simulink model "FSAC2021_V1"  (R2014a)
settings: Solver=FixedStepDiscrete  StartTime=0.0  StopTime=inf  FixedStep=0.0005  RelTol=1e-3
model workspace (MAT data in the model file):
  AS_READY = Simulink.Parameter
  AS_READY.Value = 2
  AS_READY.DataType = 'uint8'
  AS_DRIVING = Simulink.Parameter
  AS_DRIVING.Value = 3
  AS_DRIVING.DataType = 'uint8'
  AS_OFF = Simulink.Parameter
  AS_OFF.Value = 1
  AS_OFF.DataType = 'uint8'
  AS_FINISH = Simulink.Parameter
  AS_FINISH.Value = 4
  AS_FINISH.DataType = 'uint8'
  AS_EMERGENCY = Simulink.Parameter
  AS_EMERGENCY.Value = 5
  AS_EMERGENCY.DataType = 'uint8'
  ENABLE = Simulink.Parameter
  ENABLE.Value = 1
  ENABLE.DataType = 'uint8'
  DISABLE = Simulink.Parameter
  DISABLE.Value = 0
  DISABLE.DataType = 'uint8'
  Tire_Radius = Simulink.Parameter
  Tire_Radius.Value = 234
  Tire_Radius.DataType = 'single'
  Ts = Simulink.Parameter
  Ts.Value = 0.0005
  Ts.DataType = 'double'
  Filter_Factor = Simulink.Parameter
  Filter_Factor.Value = 0.5
  Filter_Factor.DataType = 'single'
  Teeth_Wheel = Simulink.Parameter
  Teeth_Wheel.Value = 60
  Teeth_Wheel.DataType = 'uint8'
  BLINK = Simulink.Parameter
  BLINK.Value = 2
  BLINK.DataType = 'uint8'
  OFF = Simulink.Parameter
  OFF.Value = 0
  OFF.DataType = 'uint8'
  ON = Simulink.Parameter
  ON.Value = 1
  ON.DataType = 'uint8'
  EBS_DISABLE = Simulink.Parameter
  EBS_DISABLE.Value = 0
  EBS_DISABLE.DataType = 'uint8'
  EBS_ARMED = Simulink.Parameter
  EBS_ARMED.Value = 1
  EBS_ARMED.DataType = 'uint8'
  EBS_ENABLE = Simulink.Parameter
  EBS_ENABLE.Value = 2
  EBS_ENABLE.DataType = 'uint8'
  MANUAL_DRIVING = Simulink.Parameter
  MANUAL_DRIVING.Value = 6
  MANUAL_DRIVING.DataType = 'uint8'
  MANUAL_MODE = Simulink.Parameter
  MANUAL_MODE.Value = 6
  MANUAL_MODE.DataType = 'uint8'
  BUZZER_START = 1
  BUZZER_EBS = Simulink.Parameter
  BUZZER_EBS.Value = 2
  BUZZER_EBS.DataType = 'uint8'
  TRACKDRIVE = Simulink.Parameter
  TRACKDRIVE.Value = 3
  TRACKDRIVE.DataType = 'uint8'
  Self_Learn_Diff = Simulink.Parameter
  Self_Learn_Diff.Value = 150
  Self_Learn_Diff.DataType = 'uint16'
  Acc_Left_Full_mv = Simulink.Parameter
  Acc_Left_Full_mv.Value = 2000
  Acc_Left_Full_mv.DataType = 'single'
  Acc_Right_Full_mv = Simulink.Parameter
  Acc_Right_Full_mv.Value = 2000
  Acc_Right_Full_mv.DataType = 'single'
  Brk_Calib_Value = Simulink.Parameter
  Brk_Calib_Value.Value = 150
  Brk_Calib_Value.DataType = 'single'
  Brk_Use_Range = Simulink.Parameter
  Brk_Use_Range.Value = 1500
  Brk_Use_Range.DataType = 'single'
  Armed = Simulink.Parameter
  Armed.Value = 1
  Armed.DataType = 'uint8'
  Enable = Simulink.Parameter
  Enable.Value = 2
  Enable.DataType = 'uint8'
  Disable = Simulink.Parameter
  Disable.Value = 0
  Disable.DataType = 'uint8'
  High_V = Simulink.Parameter
  High_V.Value = 60
  High_V.DataType = 'uint8'
  reg_num = Simulink.Parameter
  reg_num.Value = 1
  reg_num.DataType = 'uint8'
  Acc_Diff = Simulink.Parameter
  Acc_Diff.Value = 0.3
  Acc_Diff.DataType = 'single'
  Mtr_Cabli = Simulink.Parameter
  Mtr_Cabli.Value = 3
  Mtr_Cabli.DataType = 'single'
  BMS_Cabli = Simulink.Parameter
  BMS_Cabli.Value = 3
  BMS_Cabli.DataType = 'single'
  EBS_Cabli = Simulink.Parameter
  EBS_Cabli.Value = 3.3
  EBS_Cabli.DataType = 'single'
  Acc_Right_Factor = Simulink.Parameter
  Acc_Right_Factor.Value = -0.0833
  Acc_Right_Factor.DataType = 'double'
  Acc_Left_Factor = Simulink.Parameter
  Acc_Left_Factor.Value = 0.045
  Acc_Left_Factor.DataType = 'double'
  Acc_Lft_Offset = Simulink.Parameter
  Acc_Lft_Offset.Value = -90
  Acc_Lft_Offset.DataType = 'int8'
  Acc_Right_Offset = Simulink.Parameter
  Acc_Right_Offset.Value = 408.33
  Acc_Right_Offset.DataType = 'single'
  RTeeth_Wheel = Simulink.Parameter
  RTeeth_Wheel.Value = 30
  RTeeth_Wheel.DataType = 'uint8'
  FTeeth_Wheel = Simulink.Parameter
  FTeeth_Wheel.Value = 60
  FTeeth_Wheel.DataType = 'uint8'
  Brk_Liquid_Prs_Offset = Simulink.Parameter
  Brk_Liquid_Prs_Offset.Value = 0
  Brk_Liquid_Prs_Offset.DataType = 'single'
  Brk_Liquid_Prs_Factor = Simulink.Parameter
  Brk_Liquid_Prs_Factor.Value = 0.001
  Brk_Liquid_Prs_Factor.DataType = 'double'
  EBS_Prs_Factor = Simulink.Parameter
  EBS_Prs_Factor.Value = 0.000303
  EBS_Prs_Factor.DataType = 'double'
  EBS_Prs_Offset = Simulink.Parameter
  EBS_Prs_Offset.Value = 0
  EBS_Prs_Offset.DataType = 'single'
  Mtr_Volt_Factor = Simulink.Parameter
  Mtr_Volt_Factor.Value = 33.33
  Mtr_Volt_Factor.DataType = 'single'
  Mtr_Volt_Offset = Simulink.Parameter
  Mtr_Volt_Offset.Value = 0
  Mtr_Volt_Offset.DataType = 'single'
  BMS_Output_Volt_Factor = Simulink.Parameter
  BMS_Output_Volt_Factor.Value = 33.33
  BMS_Output_Volt_Factor.DataType = 'single'
  BMS_Output_Volt_Offset = Simulink.Parameter
  BMS_Output_Volt_Offset.Value = 0
  BMS_Output_Volt_Offset.DataType = 'single'
  Min = Simulink.Parameter
  Min.Value = 10
  Min.DataType = 'uint8'
  ACC_LOCK_UPSET = Simulink.Parameter
  ACC_LOCK_UPSET.Value = 25
  ACC_LOCK_UPSET.DataType = 'uint8'
  BRK_DISPSENS_LOWLIMIT = Simulink.Parameter
  BRK_DISPSENS_LOWLIMIT.Value = 2
  BRK_DISPSENS_LOWLIMIT.DataType = 'single'
  BRK_ENGAGED = Simulink.Parameter
  BRK_ENGAGED.Value = 1
  BRK_ENGAGED.DataType = 'uint8'
  BRK_Engaged_Angle = Simulink.Parameter
  BRK_Engaged_Angle.Value = 8
  BRK_Engaged_Angle.DataType = 'double'
  BRK_MOVE = Simulink.Parameter
  BRK_MOVE.Value = 3
  BRK_MOVE.DataType = 'uint8'
  BRK_MTR_RATIO = Simulink.Parameter
  BRK_MTR_RATIO.Value = 10
  BRK_MTR_RATIO.DataType = 'uint8'
  BRK_TOZERO = Simulink.Parameter
  BRK_TOZERO.Value = 2
  BRK_TOZERO.DataType = 'uint8'
  Brake = 11
  Brk_Pct2Angle = Simulink.Parameter
  Brk_Pct2Angle.Value = 0.9
  Brk_Pct2Angle.DataType = 'single'
  Brk_Prop2Angle = Simulink.Parameter
  Brk_Prop2Angle.Value = 1
  Brk_Prop2Angle.DataType = 'single'
  DIFF_RATIO = Simulink.Parameter
  DIFF_RATIO.Value = 5
  DIFF_RATIO.DataType = 'uint8'
  DISABLE1 = Simulink.Parameter
  DISABLE1.Value = 0
  DISABLE1.DataType = 'uint8'
  ENABLE1 = Simulink.Parameter
  ENABLE1.Value = 1
  ENABLE1.DataType = 'uint8'
  MANUAL_MODEL = Simulink.Parameter
  MANUAL_MODEL.Value = 6
  MANUAL_MODEL.DataType = 'uint8'
  PULSES_PER_CIRCLE = Simulink.Parameter
  PULSES_PER_CIRCLE.Value = 6400
  PULSES_PER_CIRCLE.DataType = 'auto'
  Pct2Kmh = Simulink.Parameter
  Pct2Kmh.Value = 0.2
  Pct2Kmh.DataType = 'double'
  Sensor_Acc_b = 101.85
  Sensor_Acc_k = -0.0185
  Str_Sen_Orig_Angle = -341
  TIRE_D = Simulink.Parameter
  TIRE_D.Value = 0.47
  TIRE_D.DataType = 'double'
  Tire_D = 0.47
  T = 0.05
libraries: simulink x189, ec55xxlib x135
(part 1 of 9)
settings Model: Creator=zxj  LastModifiedBy=zxj
settings OptimizationCC: InlineParams=on  InlineInvariantSignals=on  RollThreshold=9  StateBitsets=on  DataBitsets=on  UseTempVars=on  ZeroExternalMemoryAtStartup=off  ZeroInternalMemoryAtStartup=off  EfficientFloat2IntCast=on  OptimizeModelRefInitCode=on  LifeSpan=1
settings DebuggingCC: InheritedTsInSrcMsg=none  ParameterOverflowMsg=none
settings HardwareCC: ProdLargestAtomicInteger=Long  ProdLargestAtomicFloat=Double  ProdIntDivRoundTo=Zero  ProdEndianess=BigEndian  ProdHWDeviceType=Freescale MPC5500
settings RTWCC: SystemTargetFile=ec55xx.tlc  MakeCommand=make_rtw optimized_fixed_point=1  GenerateMakefile=off  TemplateMakefile=ec55xx_lcc.tmf  PostCodeGenCommand=ec55xx_pst_s2(buildInfo)  Description=Target for EC55XX  GenerateReport=on  ProcessScript=ec55xx_make_rtw_hook  IncludeHyperlinkInReport=on  LaunchReport=on
settings CodeAppCC: IgnoreCustomStorageClasses=off
settings STFCustomTargetCC: ModelReferenceCompliant=off  ConcurrentExecutionCompliant=off  IncludeMdlTerminateFcn=off  GeneratePreprocessorConditionals=Use local settings  CombineOutputUpdateFcns=on  SuppressErrorStatus=on  ERTCustomFileBanners=on  SupportContinuousTime=off  SupportNonInlinedSFcns=off  MATLABClassNameForMDSCustomization=Simulink.SoftwareTarget.ERTCustomization  GRTInterface=off  SystemTargetFile=ec55xx.tlc
settings ERTTargetCC: GenerateSampleERTMain=off  ModelReferenceCompliant=off  IncludeMdlTerminateFcn=off  SuppressErrorStatus=on  GenerateASAP2=on  ERTSrcFileBannerTemplate=ec55xx_code_template.cgt  ERTHdrFileBannerTemplate=ec55xx_code_template.cgt  ERTDataSrcFileTemplate=ec55xx_code_template.cgt  ERTDataHdrFileTemplate=ec55xx_code_template.cgt  ERTCustomFileTemplate=ec55xx_file_process.tlc

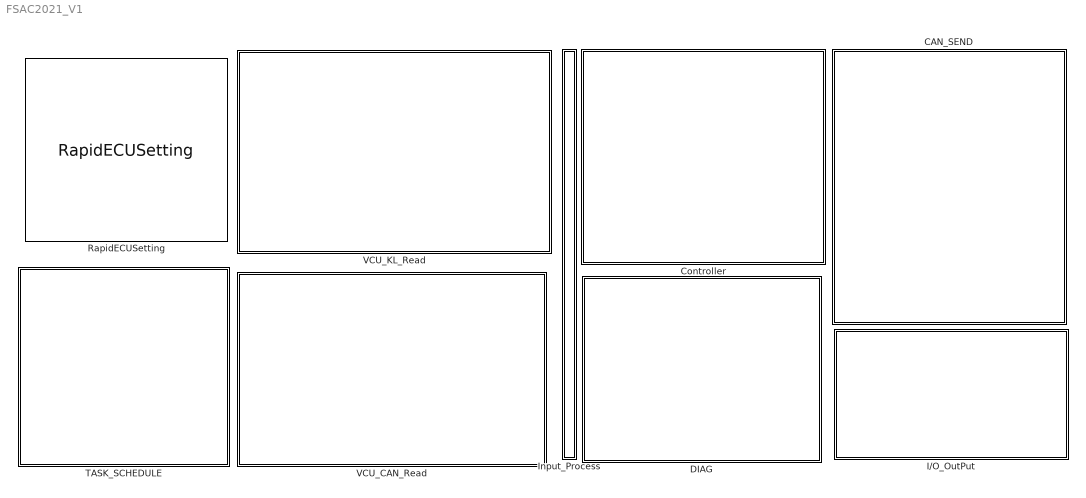
== system FSAC2021_V1 ==
  CAN_SEND : Subsystem
  Controller : Subsystem
  DIAG : Subsystem
  I/O_OutPut : Subsystem
  Input_Process : Subsystem
  RapidECUSetting : ec55xxlib/RapidECU_U2/RapidECUSetting
      link override CAN: bcmt=Extended(29-bit ID)
      link override RTI: rtiperiod=0.0005
  TASK_SCHEDULE : Subsystem
  VCU_CAN_Read : Subsystem
  VCU_KL_Read : Subsystem

== system FSAC2021_V1/CAN_SEND ==
  (BRK、STR、DRIVER) : Subsystem  SystemSampleTime=0.05
  From21 : From  Commented=on  GotoTag=Brk_Mtr_Enable_funCall  TagVisibility=global
  Rate Transition{1..19} (19 alike) : RateTransition  Deterministic=off
  Subsystem1 : Subsystem
  Subsystem2 : Subsystem
  Subsystem3 : Subsystem
  Unit Delay{1..6} (6 alike) : UnitDelay  SampleTime=-1
  wires:
  [enable_operation_ctrl] -> Rate Transition4/1
  [new_set_pint_ctrl] -> Rate Transition5/1
  [abs_or_rel_ctrl] -> Rate Transition6/1
  [halt_ctrl] -> Rate Transition8/1
  [quick_stop_ctrl] -> Rate Transition3/1
  [enable_voltage_ctrl] -> Rate Transition2/1
  [position_set] -> Rate Transition9/1
  [switch_on_ctrl] -> Rate Transition1/1
  [nmt_nodeorder] -> Rate Transition11/1
  [nmt_nodectrl] -> Rate Transition12/1
  [encoder_msg_data] -> Rate Transition15/1
  Rate Transition10/1 -> Unit Delay5/1
  [BatVoltage_Out] -> Rate Transition10/1
  Rate Transition13/1 -> Unit Delay1/1
  Rate Transition14/1 -> Unit Delay2/1
  [Motor_Current_Speed] -> Rate Transition13/1
  [ASSI_State] -> Rate Transition14/1
  [Vel_Spd] -> Rate Transition16/1
  Rate Transition16/1 -> Unit Delay6/1
  [Fault_Reset] -> Rate Transition7/1
  Rate Transition7/1 -> Subsystem1/15(Fault_Reset)
  Rate Transition15/1 -> Subsystem1/14(Encoder_Msg_Data)
  [tmtsdocan] -> Subsystem1/13(Tmt_SDO_CAN_FunCall)
  [tmtnnmtcan] -> Subsystem1/10(Tmt_NMT_CAN_FunCall)
  Rate Transition11/1 -> Subsystem1/11(NMT_nodeorder)
  Rate Transition12/1 -> Subsystem1/12(NMT_nodectrl)
  [tmprdo1can] -> Subsystem1/1(Tmt_RPD01_CAN_FunCall)
  Rate Transition1/1 -> Subsystem1/2(Switch_On_Ctrl)
  Rate Transition6/1 -> Subsystem1/7(Abs_or_Rel_Ctrl)
  Rate Transition3/1 -> Subsystem1/4(Quick_Stop_Ctrl)
  Rate Transition2/1 -> Subsystem1/3(Enable_Voltage_Ctrl)
  Rate Transition4/1 -> Subsystem1/5(Enable_Operation_Ctrl)
  Rate Transition5/1 -> Subsystem1/6(New_Set_Point_Ctrl)
  Rate Transition8/1 -> Subsystem1/8(Halt_Ctrl)
  Rate Transition9/1 -> Subsystem1/9(Position_set)
  Unit Delay1/1 -> (BRK、STR、DRIVER)/2(Motor_Current_Speed)
  Unit Delay2/1 -> (BRK、STR、DRIVER)/3(ASSI_State)
  Unit Delay5/1 -> (BRK、STR、DRIVER)/1(BatVoltage_Out)
  Unit Delay6/1 -> (BRK、STR、DRIVER)/4(vspd)
  [ASSI_State] -> Rate Transition19/1
  Rate Transition19/1 -> Subsystem1/16(ASSI_STATE)
  [FunCall_50ms_Duty11] -> Subsystem2/Trigger
  [Brk_Mtr_GoalPos] -> Rate Transition17/1
  [Acc_Ctr] -> Rate Transition18/1
  Rate Transition17/1 -> Unit Delay3/1
  Rate Transition18/1 -> Unit Delay4/1
  Unit Delay4/1 -> Subsystem2/2(Acc_Cmd)
  Unit Delay3/1 -> Subsystem2/1(Brk_Mtr_GoalPos)
  [FunCall_30ms_Duty] -> (BRK、STR、DRIVER)/Trigger

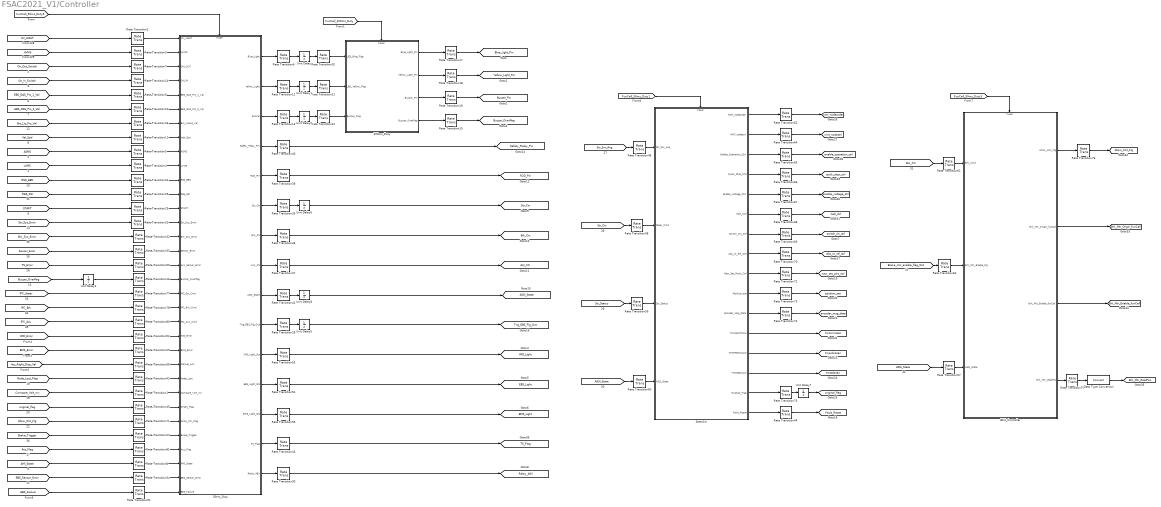
== system FSAC2021_V1/Controller ==
  200ms_Duty : Subsystem
  50ms_Duty : Subsystem
  BCU_Controller : Subsystem
  Data Type Conversion : DataTypeConversion
  Rate Transition{1..37,39..46,50..81} (77 alike) : RateTransition  Deterministic=off
  SteerCtr : Subsystem
  Unit Delay{,1..3,5..8} (8 alike) : UnitDelay  SampleTime=-1
  tag scope: ASSI_State=global, Acc_Ctr=global, Allow_Ctrl_Flg=global, BMS_Light=global, Blue_Light_Pin=global, Brk_Ctr=global, Brk_Mtr_Enable_funCall=global, Brk_Mtr_GoalPos=global, Brk_Mtr_Origin_funCall=global, Buzzer_Overflag=global, Buzzer_Pin=global, EBS_Light=global, Fault_Reset=global, IMD_Light=global, R2D_Pin=global, Relay_48V=global, Safety_Relay_Pin=global, Str_Ctr=global, TS_Flag=global, Trig_EBS_Flg_Out=global, Yellow_Light_Pin=global, abs_or_rel_ctrl=global, enable_operation_ctrl=global, enable_voltage_ctrl=global, encoder_msg_data=global, halt_ctrl=global, new_set_pint_ctrl=global, nmt_nodectrl=global, nmt_nodeorder=global, original_flag=global, position_set=global, quick_stop_ctrl=global, switch_on_ctrl=global, tmprdo1can=global, tmtnnmtcan=global, tmtsdocan=global
  wires:
  [On_Out_Switch] -> Rate Transition7/1
  [ASMS] -> Rate Transition5/1
  [AMI_State] -> Rate Transition8/1
  [EBS_GAS_Prs_2_Val] -> Rate Transition10/1
  [EBS_GAS_Prs_1_Val] -> Rate Transition9/1
  [HVMS] -> Rate Transition3/1
  Rate Transition8/1 -> 50ms_Duty/31(AMI_State)
  Rate Transition4/1 -> 50ms_Duty/10(LVMS)
  [LVMS] -> Rate Transition4/1
  Rate Transition10/1 -> 50ms_Duty/6(EBS_GAS_Prs_2_Val)
  Rate Transition7/1 -> 50ms_Duty/3(ON_OUT)
  [HV_LIGHT] -> Rate Transition2/1
  Rate Transition3/1 -> 50ms_Duty/2(HVMS)
  Rate Transition11/1 -> 50ms_Duty/8(Veh_Spd)
  Rate Transition2/1 -> 50ms_Duty/1(HV_LIGHT)
  [Vel_Spd] -> Rate Transition11/1
  Rate Transition9/1 -> 50ms_Duty/5(EBS_GAS_Prs_1_Val)
  Rate Transition5/1 -> 50ms_Duty/9(ASMS)
  [FunCall_50ms_Duty5] -> 50ms_Duty/Trigger
  [FunCall_200ms_Duty] -> 200ms_Duty/Trigger
  Rate Transition6/1 -> Unit Delay/1
  Rate Transition12/1 -> Unit Delay1/1
  Rate Transition13/1 -> Unit Delay2/1
  50ms_Duty/1(Blue_Light) -> Rate Transition6/1
  50ms_Duty/2(Yellow_Light) -> Rate Transition12/1
  50ms_Duty/3(Buzzer) -> Rate Transition13/1
  Unit Delay3/1 -> Rate Transition16/1
  Unit Delay/1 -> Rate Transition20/1
  Unit Delay1/1 -> Rate Transition21/1
  Unit Delay2/1 -> Rate Transition22/1
  [On_In_Switch] -> Rate Transition14/1
  Rate Transition14/1 -> 50ms_Duty/4(ON_IN)
  Rate Transition16/1 -> 50ms_Duty/18(Buzzer_Overflag)
  200ms_Duty/1(Blue_Light_Pin) -> Rate Transition17/1
  200ms_Duty/2(Yellow_Light_Pin) -> Rate Transition18/1
  200ms_Duty/3(Buzzer_Pin) -> Rate Transition19/1
  Rate Transition17/1 -> [Blue_Light_Pin]
  Rate Transition18/1 -> [Yellow_Light_Pin]
  Rate Transition19/1 -> [Buzzer_Pin]
  Rate Transition20/1 -> 200ms_Duty/1(LED_Blue_Flag)
  Rate Transition21/1 -> 200ms_Duty/2(LED_Yellow_Flag)
  Rate Transition22/1 -> 200ms_Duty/3(Buzzer_Flag)
  [START] -> Rate Transition23/1
  Rate Transition23/1 -> 50ms_Duty/13(START)
  [RES_EBS] -> Rate Transition24/1
  Rate Transition24/1 -> 50ms_Duty/11(RES_EBS)
  [RES_GO] -> Rate Transition25/1
  Rate Transition25/1 -> 50ms_Duty/12(RES_GO)
  Rate Transition26/1 -> 50ms_Duty/7(Brk_Liquid_Val)
  [Brs_Liq_Prs_Val] -> Rate Transition26/1
  200ms_Duty/4(Buzzer_Overflag) -> Rate Transition15/1
  Rate Transition15/1 -> [Buzzer_Overflag]
  [Buzzer_Overflag] -> Unit Delay3/1
  [Str_Sys_Error] -> Rate Transition31/1
  [Brk_Sys_Error] -> Rate Transition32/1
  [Sensor_Error] -> Rate Transition33/1
  Rate Transition31/1 -> 50ms_Duty/14(Str_Sys_Error)
  Rate Transition32/1 -> 50ms_Duty/15(Brk_Sys_Error)
  Rate Transition33/1 -> 50ms_Duty/16(Sensor_Error)
  50ms_Duty/6(Str_Ctr) -> Rate Transition35/1
  50ms_Duty/7(Brk_Ctr) -> Rate Transition36/1
  50ms_Duty/8(Acc_Ctr) -> Rate Transition37/1
  Rate Transition35/1 -> Unit Delay6/1
  Rate Transition36/1 -> [Brk_Ctr]
  Rate Transition37/1 -> [Acc_Ctr]
  Rate Transition39/1 -> [R2D_Pin]
  50ms_Duty/5(R2D_Pin) -> Rate Transition39/1
  50ms_Duty/4(Safety_Relay_Pin) -> Rate Transition40/1
  Rate Transition40/1 -> [Safety_Relay_Pin]
  50ms_Duty/9(ASSI_State) -> Rate Transition41/1
  Rate Transition41/1 -> Unit Delay8/1
  [Node_Lost_Flag] -> Rate Transition42/1
  Rate Transition42/1 -> 50ms_Duty/25(Node_Lost)
  [TS_Error] -> Rate Transition50/1
  Rate Transition50/1 -> 50ms_Duty/17(Acc_Sensor_Error)
  50ms_Duty/10(Trig_EBS_Flg_Out) -> Rate Transition28/1
  Rate Transition28/1 -> Unit Delay5/1
  Unit Delay5/1 -> [Trig_EBS_Flg_Out]
  [BMS_Error] -> Rate Transition29/1
  Rate Transition29/1 -> 50ms_Duty/23(BMS_Error)
  Rate Transition52/1 -> 50ms_Duty/22(IMD_Error)
  [IMD_Error] -> Rate Transition52/1
  50ms_Duty/11(IMD_Light_Sts) -> Rate Transition53/1
  50ms_Duty/12(EBS_Light_Sts) -> Rate Transition54/1
  50ms_Duty/13(BMS_Light_Sts) -> Rate Transition55/1
  Rate Transition53/1 -> [IMD_Light]
  Rate Transition54/1 -> [EBS_Light]
  Rate Transition55/1 -> [BMS_Light]
  Rate Transition56/1 -> 50ms_Duty/24(Manual_Acc)
  [Acc_Right_Disp_Val] -> Rate Transition56/1
  SteerCtr/9(New_Set_Point_Ctrl) -> Rate Transition72/1
  SteerCtr/10(Position_set) -> Rate Transition73/1
  SteerCtr/11(Encoder_Msg_Data) -> Rate Transition74/1
  SteerCtr/2(NMT_nodectrl) -> Rate Transition64/1
  SteerCtr/3(Enable_Operation_Ctrl) -> Rate Transition65/1
  SteerCtr/4(Quick_Stop_Ctrl) -> Rate Transition66/1
  SteerCtr/5(Enable_Voltage_Ctrl) -> Rate Transition67/1
  SteerCtr/6(Halt_Ctrl) -> Rate Transition68/1
  SteerCtr/7(Switch_On_Ctrl) -> Rate Transition69/1
  SteerCtr/8(Abs_or_Rel_Ctrl) -> Rate Transition70/1
  SteerCtr/1(NMT_nodeorder) -> Rate Transition62/1
  [Str_Ctr] -> Rate Transition58/1
  [Str_Status] -> Rate Transition59/1
  [ASSI_State] -> Rate Transition60/1
  [Brk_Ctr] -> Rate Transition61/1
  [Brake_mtr_enable_flag_Out] -> Rate Transition63/1
  BCU_Controller/1(Allow_Ctrl_Flg) -> Rate Transition76/1
  BCU_Controller/4(Brk_Mtr_GoalPos) -> Rate Transition79/1
  Data Type Conversion/1 -> [Brk_Mtr_GoalPos]
  Rate Transition58/1 -> SteerCtr/2(Steer_Cmd)
  Rate Transition59/1 -> SteerCtr/3(Str_Status)
  Rate Transition60/1 -> SteerCtr/4(ASSI_State)
  Rate Transition61/1 -> BCU_Controller/1(Brk_Cmd)
  Rate Transition63/1 -> BCU_Controller/2(Brk_Mtr_Enable_Flg)
  Rate Transition62/1 -> [nmt_nodeorder]
  Rate Transition64/1 -> [nmt_nodectrl]
  Rate Transition65/1 -> [enable_operation_ctrl]
  Rate Transition66/1 -> [quick_stop_ctrl]
  Rate Transition67/1 -> [enable_voltage_ctrl]
  Rate Transition68/1 -> [halt_ctrl]
  Rate Transition69/1 -> [switch_on_ctrl]
  Rate Transition70/1 -> [abs_or_rel_ctrl]
  Rate Transition72/1 -> [new_set_pint_ctrl]
  Rate Transition73/1 -> [position_set]
  Rate Transition74/1 -> [encoder_msg_data]
  SteerCtr/15(Original_Flag) -> Rate Transition75/1
  Rate Transition76/1 -> [Allow_Ctrl_Flg]
  BCU_Controller/2(Brk_Mtr_Origin_funCall) -> [Brk_Mtr_Origin_funCall]
  BCU_Controller/3(Brk_Mtr_Enable_funCall) -> [Brk_Mtr_Enable_funCall]
  Rate Transition79/1 -> Data Type Conversion/1
  Rate Transition75/1 -> Unit Delay7/1
  SteerCtr/12(TmtNNMTCAN) -> [tmtnnmtcan]
  SteerCtr/13(TmtRPDO1CAN) -> [tmprdo1can]
  SteerCtr/14(TmtSDOCAN) -> [tmtsdocan]
  [FunCall_50ms_Duty1] -> SteerCtr/Trigger
  [FunCall_50ms_Duty3] -> BCU_Controller/Trigger
  Rate Transition1/1 -> 50ms_Duty/26(Compare_Volt_mv)
  [Compare_Volt_mv] -> Rate Transition1/1
  50ms_Duty/14(TS_Flag) -> Rate Transition43/1
  Rate Transition43/1 -> [TS_Flag]
  Unit Delay7/1 -> [original_flag]
  SteerCtr/16(Fault_Reset) -> Rate Transition44/1
  Rate Transition44/1 -> [Fault_Reset]
  Unit Delay6/1 -> [Str_Ctr]
  Rate Transition45/1 -> 50ms_Duty/27(Origin_Flag)
  [original_flag] -> Rate Transition45/1
  [Str_Snr_Ang] -> Rate Transition46/1
  Rate Transition46/1 -> SteerCtr/1(Str_Snr_Ang)
  [ASSI_State] -> Rate Transition57/1
  Rate Transition57/1 -> BCU_Controller/3(ASSI_State)
  Rate Transition71/1 -> 50ms_Duty/28(Allow_Ctr_Flag)
  [Allow_Ctrl_Flg] -> Rate Transition71/1
  [IPC_Steer] -> Rate Transition77/1
  [IPC_Acc] -> Rate Transition80/1
  [IPC_Brk] -> Rate Transition78/1
  Rate Transition77/1 -> 50ms_Duty/19(IPC_Str_Cmd)
  Rate Transition78/1 -> 50ms_Duty/20(IPC_Brk_Cmd)
  Rate Transition80/1 -> 50ms_Duty/21(IPC_Acc_Cmd)
  Rate Transition27/1 -> 50ms_Duty/29("Brake_Trigger ")
  [Brake_Trigger] -> Rate Transition27/1
  Rate Transition81/1 -> 50ms_Duty/30(Acc_Flag)
  [Acc_Flag] -> Rate Transition81/1
  Rate Transition34/1 -> 50ms_Duty/32(EBS_Sensor_Error)
  [EBS_Sensor_Error] -> Rate Transition34/1
  Unit Delay8/1 -> [ASSI_State]
  50ms_Duty/15(Relay_48V) -> Rate Transition30/1
  Rate Transition30/1 -> [Relay_48V]
  [EBS_Failure] -> Rate Transition51/1
  Rate Transition51/1 -> 50ms_Duty/33(EBS_Failure)

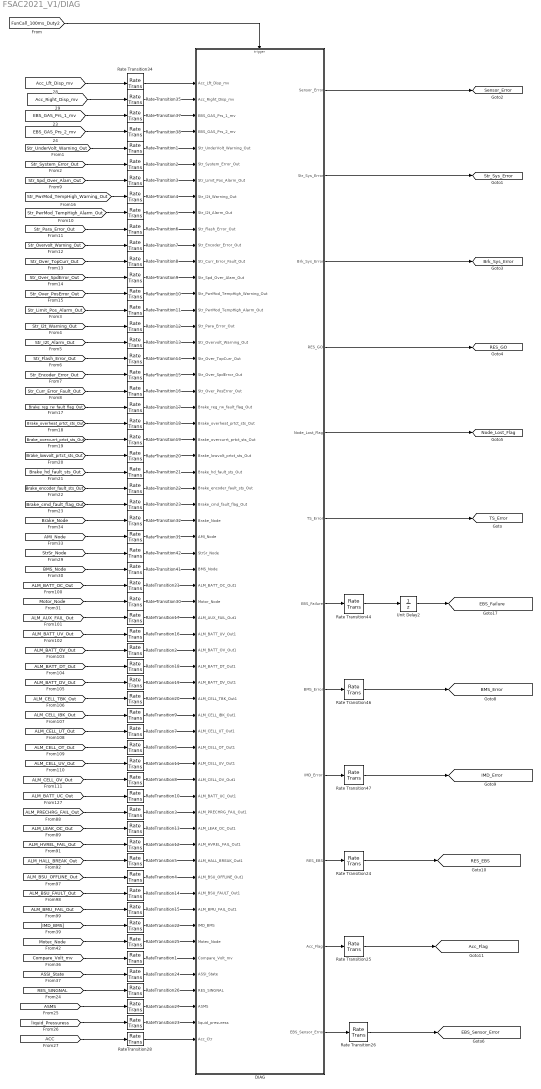
== system FSAC2021_V1/DIAG ==
  DIAG : Subsystem
  Rate Transition{1..26,30..32,34..35,37..38,41..42,44,46..47} (38 alike) : RateTransition  Deterministic=off
  RateTransition{1..28} (28 alike) : RateTransition
  Unit Delay2 : UnitDelay  SampleTime=-1
  tag scope: Acc_Flag=global, BMS_Error=global, Brk_Sys_Error=global, EBS_Failure=global, EBS_Sensor_Error=global, IMD_Error=global, Node_Lost_Flag=global, RES_EBS=global, RES_GO=global, Sensor_Error=global, Str_Sys_Error=global, TS_Error=global
  wires:
  Rate Transition35/1 -> DIAG/2(Acc_Right_Disp_mv)
  Rate Transition37/1 -> DIAG/3(EBS_GAS_Prs_1_mv)
  Rate Transition38/1 -> DIAG/4(EBS_GAS_Prs_2_mv)
  Rate Transition34/1 -> DIAG/1(Acc_Lft_Disp_mv)
  [Acc_Lft_Disp_mv] -> Rate Transition34/1
  [EBS_GAS_Prs_1_mv] -> Rate Transition37/1
  [EBS_GAS_Prs_2_mv] -> Rate Transition38/1
  [Acc_Right_Disp_mv] -> Rate Transition35/1
  [FunCall_100ms_Duty2] -> DIAG/Trigger
  [Str_UnderVolt_Warning_Out] -> Rate Transition1/1
  [Str_System_Error_Out] -> Rate Transition2/1
  [Str_Spd_Over_Alam_Out] -> Rate Transition3/1
  [Str_PwrMod_TempHigh_Warning_Out] -> Rate Transition4/1
  [Str_PwrMod_TempHigh_Alarm_Out] -> Rate Transition5/1
  [Str_Para_Error_Out] -> Rate Transition6/1
  [Str_Overvolt_Warning_Out] -> Rate Transition7/1
  [Str_Over_TopCurr_Out] -> Rate Transition8/1
  [Str_Over_SpdError_Out] -> Rate Transition9/1
  [Str_Over_PosError_Out] -> Rate Transition10/1
  [Str_Limit_Pos_Alarm_Out] -> Rate Transition11/1
  [Str_I2t_Warning_Out] -> Rate Transition12/1
  [Str_I2t_Alarm_Out] -> Rate Transition13/1
  [Str_Flash_Error_Out] -> Rate Transition14/1
  [Str_Encoder_Error_Out] -> Rate Transition15/1
  [Str_Curr_Error_Fault_Out] -> Rate Transition16/1
  Rate Transition1/1 -> DIAG/5(Str_UnderVolt_Warning_Out)
  Rate Transition2/1 -> DIAG/6(Str_System_Error_Out)
  Rate Transition3/1 -> DIAG/7(Str_Limit_Pos_Alarm_Out)
  Rate Transition4/1 -> DIAG/8(Str_I2t_Warning_Out)
  Rate Transition5/1 -> DIAG/9(Str_I2t_Alarm_Out)
  Rate Transition6/1 -> DIAG/10(Str_Flash_Error_Out)
  Rate Transition7/1 -> DIAG/11(Str_Encoder_Error_Out)
  Rate Transition8/1 -> DIAG/12(Str_Curr_Error_Fault_Out)
  Rate Transition9/1 -> DIAG/13(Str_Spd_Over_Alam_Out)
  Rate Transition10/1 -> DIAG/14(Str_PwrMod_TempHigh_Warning_Out)
  Rate Transition11/1 -> DIAG/15(Str_PwrMod_TempHigh_Alarm_Out)
  Rate Transition12/1 -> DIAG/16(Str_Para_Error_Out)
  Rate Transition13/1 -> DIAG/17(Str_Overvolt_Warning_Out)
  Rate Transition15/1 -> DIAG/19(Str_Over_SpdError_Out)
  Rate Transition14/1 -> DIAG/18(Str_Over_TopCurr_Out)
  Rate Transition16/1 -> DIAG/20(Str_Over_PosError_Out)
  DIAG/1(Sensor_Error) -> [Sensor_Error]
  DIAG/2(Str_Sys_Error) -> [Str_Sys_Error]
  [Brake_overcurrt_prtct_sts_Out] -> Rate Transition19/1
  [Brake_overheat_prtct_sts_Out] -> Rate Transition18/1
  [Brake_reg_rw_fault_flag_Out] -> Rate Transition17/1
  [Brake_cmd_fault_flag_Out] -> Rate Transition23/1
  [Brake_hd_fault_sts_Out] -> Rate Transition21/1
  [Brake_encoder_fault_sts_Out] -> Rate Transition22/1
  [Brake_lowvolt_prtct_sts_Out] -> Rate Transition20/1
  Rate Transition17/1 -> DIAG/21(Brake_reg_rw_fault_flag_Out)
  Rate Transition18/1 -> DIAG/22(Brake_overheat_prtct_sts_Out)
  Rate Transition19/1 -> DIAG/23(Brake_overcurrt_prtct_sts_Out)
  Rate Transition20/1 -> DIAG/24(Brake_lowvolt_prtct_sts_Out)
  Rate Transition21/1 -> DIAG/25(Brake_hd_fault_sts_Out)
  Rate Transition22/1 -> DIAG/26(Brake_encoder_fault_sts_Out)
  Rate Transition23/1 -> DIAG/27(Brake_cmd_fault_flag_Out)
  DIAG/3(Brk_Sys_Error) -> [Brk_Sys_Error]
  DIAG/4(RES_GO) -> [RES_GO]
  [Motor_Node] -> Rate Transition30/1
  [AMI_Node] -> Rate Transition31/1
  [Brake_Node] -> Rate Transition32/1
  [BMS_Node] -> Rate Transition41/1
  [StrSr_Node] -> Rate Transition42/1
  Rate Transition30/1 -> DIAG/33(Motor_Node)
  Rate Transition31/1 -> DIAG/29(AMI_Node)
  Rate Transition32/1 -> DIAG/28(Brake_Node)
  Rate Transition41/1 -> DIAG/31(BMS_Node)
  Rate Transition42/1 -> DIAG/30(StrSr_Node)
  DIAG/5(Node_Lost_Flag) -> [Node_Lost_Flag]
  DIAG/6(TS_Error) -> [TS_Error]
  DIAG/7(EBS_Failure) -> Rate Transition44/1
  Rate Transition44/1 -> Unit Delay2/1
  Unit Delay2/1 -> [EBS_Failure]
  [ALM_BATT_OV_Out] -> RateTransition2/1
  RateTransition2/1 -> DIAG/36(ALM_BATT_OV_Out1)
  [ALM_PRECHRG_FAIL_Out] -> RateTransition3/1
  RateTransition3/1 -> DIAG/46(ALM_PRECHRG_FAIL_Out1)
  [ALM_BSU_OFFLINE_Out] -> RateTransition4/1
  RateTransition4/1 -> DIAG/50(ALM_BSU_OFFLINE_Out1)
  [ALM_HALL_BREAK_Out] -> RateTransition5/1
  RateTransition5/1 -> DIAG/49(ALM_HALL_BREAK_Out1)
  [ALM_CELL_OT_Out] -> RateTransition6/1
  RateTransition6/1 -> DIAG/42(ALM_CELL_OT_Out1)
  [ALM_CELL_UT_Out] -> RateTransition7/1
  RateTransition7/1 -> DIAG/41(ALM_CELL_UT_Out1)
  [ALM_CELL_OV_Out] -> RateTransition8/1
  RateTransition8/1 -> DIAG/44(ALM_CELL_OV_Out1)
  [ALM_CELL_IBK_Out] -> RateTransition9/1
  RateTransition9/1 -> DIAG/40(ALM_CELL_IBK_Out1)
  [ALM_BATT_UC_Out] -> RateTransition10/1
  RateTransition10/1 -> DIAG/45(ALM_BATT_UC_Out1)
  [ALM_CELL_UV_Out] -> RateTransition11/1
  RateTransition11/1 -> DIAG/43(ALM_CELL_UV_Out1)
  [ALM_HVREL_FAIL_Out] -> RateTransition12/1
  RateTransition12/1 -> DIAG/48(ALM_HVREL_FAIL_Out1)
  [ALM_LEAK_OC_Out] -> RateTransition13/1
  RateTransition13/1 -> DIAG/47(ALM_LEAK_OC_Out1)
  [ALM_BSU_FAULT_Out] -> RateTransition14/1
  RateTransition14/1 -> DIAG/51(ALM_BSU_FAULT_Out1)
  [ALM_BMU_FAIL_Out] -> RateTransition15/1
  RateTransition15/1 -> DIAG/52(ALM_BMU_FAIL_Out1)
  [ALM_BATT_UV_Out] -> RateTransition16/1
  RateTransition16/1 -> DIAG/35(ALM_BATT_UV_Out1)
  [ALM_AUX_FAIL_Out] -> RateTransition17/1
  RateTransition17/1 -> DIAG/34(ALM_AUX_FAIL_Out1)
  [ALM_BATT_DT_Out] -> RateTransition18/1
  RateTransition18/1 -> DIAG/37(ALM_BATT_DT_Out1)
  [ALM_BATT_DV_Out] -> RateTransition19/1
  RateTransition19/1 -> DIAG/38(ALM_BATT_DV_Out1)
  [ALM_CELL_TBK_Out] -> RateTransition20/1
  RateTransition20/1 -> DIAG/39(ALM_CELL_TBK_Out1)
  [ALM_BATT_OC_Out] -> RateTransition21/1
  RateTransition21/1 -> DIAG/32(ALM_BATT_OC_Out1)
  DIAG/8("BMS_Error ") -> Rate Transition46/1
  Rate Transition46/1 -> [BMS_Error]
  [IMD_BMS] -> RateTransition22/1
  RateTransition22/1 -> DIAG/53("IMD_BMS ")
  DIAG/9(IMD_Error) -> Rate Transition47/1
  Rate Transition47/1 -> [IMD_Error]
  RateTransition25/1 -> DIAG/54(Motec_Node)
  [Motec_Node] -> RateTransition25/1
  RateTransition1/1 -> DIAG/55(Compare_Volt_mv)
  [Compare_Volt_mv] -> RateTransition1/1
  RateTransition24/1 -> DIAG/56(ASSI_State)
  [ASSI_State] -> RateTransition24/1
  [RES_SINGNAL] -> RateTransition26/1
  RateTransition26/1 -> DIAG/57(RES_SINGNAL)
  [ASMS] -> RateTransition27/1
  RateTransition27/1 -> DIAG/58(ASMS)
  DIAG/10(RES_EBS) -> Rate Transition24/1
  Rate Transition24/1 -> [RES_EBS]
  [liquid_Pressuress] -> RateTransition23/1
  RateTransition23/1 -> DIAG/59(liquid_presuress)
  RateTransition28/1 -> DIAG/60(Acc_Ctr)
  [ACC] -> RateTransition28/1
  DIAG/11(Acc_Flag) -> Rate Transition25/1
  Rate Transition25/1 -> [Acc_Flag]
  DIAG/12(EBS_Sensor_Error) -> Rate Transition26/1
  Rate Transition26/1 -> [EBS_Sensor_Error]

== system FSAC2021_V1/I//O_OutPut ==
  Subsystem : Subsystem
  wires:
  [Blue_Light_Pin] -> Subsystem/1(Blue_Light_Pin)
  [Yellow_Light_Pin] -> Subsystem/2(Yellow_Light_Pin)
  [Buzzer_Pin] -> Subsystem/3(Buzzer_pin)
  [Safety_Relay_Pin] -> Subsystem/4(Safety_Relay_Pin)
  [Relay_48V] -> Subsystem/5(Relay_48V_Pin)
  [R2D_Pin] -> Subsystem/6(R2D_pin)
  [IMD_Light] -> Subsystem/7(IMD_Light)
  [EBS_Light] -> Subsystem/8(EBS_Light)
  [BMS_Light] -> Subsystem/9(BMS_Light)
  [FunCall_50ms_Duty10] -> Subsystem/Trigger
  [liquid_Pressuress] -> Subsystem/10(Liquid_Pressure)

== system FSAC2021_V1/Input_Process ==
  KL_Sig_Process : Subsystem
  Rate Transition{1,3..7,9..12,14..15,18..19,21..26} (20 alike) : RateTransition  Deterministic=off
  tag scope: ACC=global, Acc_Lft_Dip_Val=global, Acc_Right_Disp_Val=global, Brs_Liq_Prs_Val=global, EBS_GAS_Prs_1_Val=global, EBS_GAS_Prs_2_Val=global, Vel_Spd=global, Whl_Spd_FF_Val=global, Whl_Spd_FL_Val=global, Whl_Spd_RL_Val=global, Whl_Spd_RR_Val=global
  wires:
  [Acc_Lft_Disp_mv] -> Rate Transition21/1
  [EBS_GAS_Prs_1_mv] -> Rate Transition14/1
  [EBS_GAS_Prs_2_mv] -> Rate Transition24/1
  [Brk_Liquid_Prs_mv] -> Rate Transition23/1
  [Acc_Right_Disp_mv] -> Rate Transition22/1
  KL_Sig_Process/1(Vel_Spd) -> Rate Transition15/1
  KL_Sig_Process/4(Whl_Spd_RL_Val) -> Rate Transition10/1
  KL_Sig_Process/2(Whl_Spd_FL_Val) -> Rate Transition12/1
  KL_Sig_Process/3(Whl_Spd_FF_Val) -> Rate Transition11/1
  Rate Transition19/1 -> KL_Sig_Process/2(FR_WhlSpd_Hz)
  KL_Sig_Process/5(Whl_Spd_RR_Val) -> Rate Transition9/1
  Rate Transition26/1 -> KL_Sig_Process/4(RR_WhlSpd_Hz)
  [RR_WhlSpd_Hz] -> Rate Transition26/1
  Rate Transition25/1 -> KL_Sig_Process/3(RL_WhlSpd_Hz)
  Rate Transition18/1 -> KL_Sig_Process/1(FL_WhlSpd_Hz)
  [RL_WhlSpd_Hz] -> Rate Transition25/1
  [FL_WhlSpd_Hz] -> Rate Transition18/1
  [FR_WhlSpd_Hz] -> Rate Transition19/1
  KL_Sig_Process/7(Acc_Right_Disp_Val) -> Rate Transition6/1
  KL_Sig_Process/6(Acc_Lft_Disp_Val) -> Rate Transition7/1
  Rate Transition24/1 -> KL_Sig_Process/9(EBS_GAS_Prs_2_mv)
  Rate Transition23/1 -> KL_Sig_Process/7(Brk_Liquid_Prs_mv)
  KL_Sig_Process/10(EBS_GAS_Prs_2_Val) -> Rate Transition3/1
  Rate Transition21/1 -> KL_Sig_Process/5(Acc_Lft_Disp_mv)
  KL_Sig_Process/8(Brk_Liquid_Prs_Val) -> Rate Transition5/1
  Rate Transition22/1 -> KL_Sig_Process/6(Acc_Right_Disp_mv)
  KL_Sig_Process/9(EBS_GAS_Prs_1_Val) -> Rate Transition4/1
  Rate Transition14/1 -> KL_Sig_Process/8(EBS_GAS_Prs_1_mv)
  [FunCall_20ms_Duty] -> KL_Sig_Process/Trigger
  Rate Transition3/1 -> [EBS_GAS_Prs_2_Val]
  Rate Transition4/1 -> [EBS_GAS_Prs_1_Val]
  Rate Transition5/1 -> [Brs_Liq_Prs_Val]
  Rate Transition6/1 -> [Acc_Right_Disp_Val]
  Rate Transition7/1 -> [Acc_Lft_Dip_Val]
  Rate Transition9/1 -> [Whl_Spd_RR_Val]
  Rate Transition10/1 -> [Whl_Spd_RL_Val]
  Rate Transition11/1 -> [Whl_Spd_FF_Val]
  Rate Transition12/1 -> [Whl_Spd_FL_Val]
  Rate Transition15/1 -> [Vel_Spd]
  KL_Sig_Process/11(ACC) -> Rate Transition1/1
  Rate Transition1/1 -> [ACC]

== system FSAC2021_V1/TASK_SCHEDULE ==
  Demux : Demux  Outputs=11
  Demux1 : Demux  Outputs=3
  Demux2 : Demux  Outputs=3
  Function-Call Generator : simulink/Ports & Subsystems/Function-Call Generator  sample_time=0.02  numberOfIterations=1
  Function-Call Generator1 : simulink/Ports & Subsystems/Function-Call Generator  sample_time=0.05  numberOfIterations=1
  Function-Call Generator2 : simulink/Ports & Subsystems/Function-Call Generator  sample_time=0.1  numberOfIterations=1
  Function-Call Generator3 : simulink/Ports & Subsystems/Function-Call Generator  sample_time=0.2  numberOfIterations=1
  Function-Call Generator4 : simulink/Ports & Subsystems/Function-Call Generator  sample_time=0.01  numberOfIterations=1
  Function-Call Generator5 : simulink/Ports & Subsystems/Function-Call Generator  sample_time=0.03  numberOfIterations=1
  tag scope: FunCall_100ms_Duty1=global, FunCall_100ms_Duty2=global, FunCall_100ms_Duty3=global, FunCall_10ms_Duty1=global, FunCall_10ms_Duty2=global, FunCall_10ms_Duty=global, FunCall_200ms_Duty=global, FunCall_20ms_Duty=global, FunCall_30ms_Duty=global, FunCall_50ms_Duty10=global, FunCall_50ms_Duty11=global, FunCall_50ms_Duty1=global, FunCall_50ms_Duty2=global, FunCall_50ms_Duty3=global, FunCall_50ms_Duty4=global, FunCall_50ms_Duty5=global, FunCall_50ms_Duty6=global, FunCall_50ms_Duty7=global, FunCall_50ms_Duty8=global, FunCall_50ms_Duty9=global
  wires:
  Function-Call Generator/1 -> [FunCall_20ms_Duty]
  Function-Call Generator1/1 -> Demux/1
  Demux/1 -> [FunCall_50ms_Duty1]
  Demux/2 -> [FunCall_50ms_Duty2]
  Demux/3 -> [FunCall_50ms_Duty3]
  Demux/5 -> [FunCall_50ms_Duty5]
  Demux/4 -> [FunCall_50ms_Duty4]
  Function-Call Generator2/1 -> Demux1/1
  Demux1/1 -> [FunCall_100ms_Duty1]
  Demux1/2 -> [FunCall_100ms_Duty2]
  Demux1/3 -> [FunCall_100ms_Duty3]
  Function-Call Generator3/1 -> [FunCall_200ms_Duty]
  Demux/6 -> [FunCall_50ms_Duty6]
  Demux/7 -> [FunCall_50ms_Duty7]
  Demux/8 -> [FunCall_50ms_Duty8]
  Demux/9 -> [FunCall_50ms_Duty9]
  Demux/10 -> [FunCall_50ms_Duty10]
  Demux/11 -> [FunCall_50ms_Duty11]
  Function-Call Generator4/1 -> Demux2/1
  Demux2/1 -> [FunCall_10ms_Duty]
  Demux2/2 -> [FunCall_10ms_Duty1]
  Demux2/3 -> [FunCall_10ms_Duty2]
  Function-Call Generator5/1 -> [FunCall_30ms_Duty]

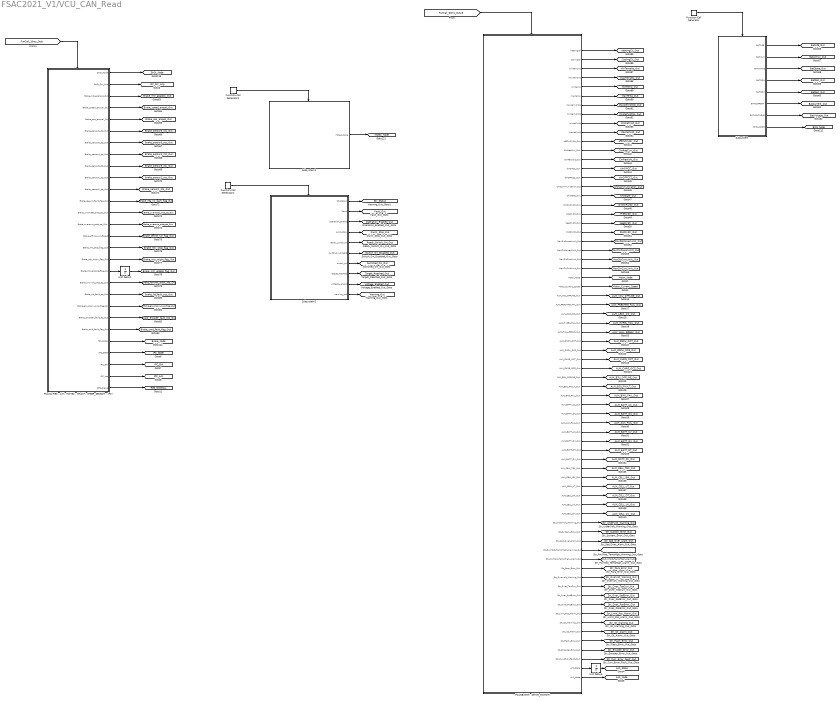
== system FSAC2021_V1/VCU_CAN_Read ==
  Function-Call Generator : simulink/Ports & Subsystems/Function-Call Generator  sample_time=0.1  numberOfIterations=1
  Function-Call Generator1 : simulink/Ports & Subsystems/Function-Call Generator  sample_time=0.5  numberOfIterations=1
  Function-Call Generator2 : simulink/Ports & Subsystems/Function-Call Generator  sample_time=0.1  numberOfIterations=1
  PCANA(RES、AMI、MOTEC、BRAKE、STEER_SENSOR、IPC) : Subsystem
  PCANB(BMS、DRIVE_MOTOR) : Subsystem
  Subsystem : Subsystem
  Subsystem1 : Subsystem
  Subsystem2 : Subsystem
  Unit Delay1 : UnitDelay  SampleTime=-1
  Unit Delay5 : UnitDelay  SampleTime=-1
  tag scope: ALM_AUX_FAIL_Out=global, ALM_BATT_DT_Out=global, ALM_BATT_DV_Out=global, ALM_BATT_OC_Out=global, ALM_BATT_OV_Out=global, ALM_BATT_UC_Out=global, ALM_BATT_UV_Out=global, ALM_BMU_FAIL_Out=global, ALM_BSU_FAULT_Out=global, ALM_BSU_OFFLINE_Out=global, ALM_CELL_IBK_Out=global, ALM_CELL_OT_Out=global, ALM_CELL_OV_Out=global, ALM_CELL_TBK_Out=global, ALM_CELL_UT_Out=global, ALM_CELL_UV_Out=global, ALM_CHRG_OCS_Out=global, ALM_CHRG_OCT_Out=global, ALM_DSCH_OCS_Out=global, ALM_DSCH_OCT_Out=global, ALM_HALL_BREAK_Out=global, ALM_HVREL_FAIL_Out=global, ALM_LEAK_OC_Out=global, ALM_PRECHRG_FAIL_Out=global, ALM_VCU_OFFLINE_Out=global, AMI_Node=global, AMI_State=global, BMS_Node=global, BatAlmLv_Out=global, BatCurrent_Out=global, BatLife_Out=global, BatSoc_Out=global, BatSoh_Out=global, BatState_Out=global, BatVoltage_Out=global, Brake_Node=global, Brake_cmd_fault_flag_Out=global, Brake_encoder_fault_sts_Out=global, Brake_go_origin_over_flag_Out=global, Brake_hd_fault_sts_Out=global, Brake_lowvolt_prtct_sts_Out=global, Brake_mtr_enable_flag_Out=global, Brake_mtr_goalpos_Out=global, Brake_mtr_origin_flag_Out=global, Brake_mtr_stop_flag_Out=global, Brake_offline_run_flag_Out=global, Brake_overcurrt_prtct_sts_Out=global, Brake_overheat_prtct_sts_Out=global, Brake_pos_enqual_Out=global, Brake_reg_rw_fault_flag_Out=global, Brake_sensor1_sts_Out=global, Brake_sensor2_sts_Out=global, Brake_sensor3_sts_Out=global, Brake_sensor4_sts_Out=global, Brake_sensor5_sts_Out=global, Brake_sensor6_sts_Out=global, Brake_speed_enqual_Out=global, ChrCommunication_Out=global, ChrReqCurr_Out=global, ChrReqVolt_Out=global, ChrState_Out=global, CoolingCtl_Out=global, Fault_Out=global, HeatingCtl_Out=global, IPC_Acc=global, IPC_Brk=global, IPC_Steer=global, MaxCellVoltNo_Out=global, MaxCellVolt_Out=global, MaxChrCurtLimit_Out=global, MaxChrPowerLimit_Out=global, MaxDisCurtLimit_Out=global, MaxDisPowerLimit_Out=global, MaxTempNo_Out=global, MaxTemp_Out=global, MinCellVoltNo_Out=global, MinCellVolt_Out=global, MinTempNo_Out=global, MinTemp_Out=global, Motec_Node=global, Motor_Current_Speed=global, Motor_Node=global, NegRlyStr_Out=global, OnChrRlyStr_Out=global, Operation_Enabled_Out=global, PosRlyStr_Out=global, PreRlyStr_Out=global, Quick_Stop_Out=global, RES_SINGNAL=global, Ready_Switch_On_Out=global, StrSr_Node=global, Str_Curr_Error_Fault_Out=global, Str_Encoder_Error_Out=global, Str_Flash_Error_Out=global, Str_I2t_Alarm_Out=global, Str_I2t_Warning_Out=global, Str_Limit_Pos_Alarm_Out=global, Str_Over_PosError_Out=global, Str_Over_SpdError_Out=global, Str_Over_TopCurr_Out=global, Str_Overvolt_Warning_Out=global, Str_Para_Error_Out=global, Str_PwrMod_TempHigh_Alarm_Out=global, Str_PwrMod_TempHigh_Warning_Out=global, Str_Snr_Ang=global, Str_Spd_Over_Alam_Out=global, Str_Status=global, Str_System_Error_Out=global, Str_UnderVolt_Warning_Out=global, Switch_On_Disabled_Out=global, Swtiched_On_Out=global, Target_Reached_Out=global, Voltage_Enabled_Out=global, Warning_Out=global, chrOFFCC2_Out=global, chrONCC_Out=global, offChrRlyStr_Out=global
  wires:
  Subsystem/1(BATLIFE) -> [BatLife_Out]
  Subsystem/2(BATALM) -> [BatAlmLv_Out]
  Subsystem/3(BATSTATE) -> [BatState_Out]
  Subsystem/4(BATSOH) -> [BatSoh_Out]
  Subsystem/5(BATSOC) -> [BatSoc_Out]
  Subsystem/6(BATCURRENT) -> [BatCurrent_Out]
  Subsystem/7(BATVOLTAGLE) -> [BatVoltage_Out]
  Function-Call Generator/1 -> Subsystem/Trigger
  Subsystem/8(BMS_NODE) -> [BMS_Node]
  PCANB(BMS、DRIVE_MOTOR)/3(mintempno) -> [MinTempNo_Out]
  PCANB(BMS、DRIVE_MOTOR)/2(coolingctl) -> [CoolingCtl_Out]
  PCANB(BMS、DRIVE_MOTOR)/4(maxtempno) -> [MaxTempNo_Out]
  PCANB(BMS、DRIVE_MOTOR)/5(mintemp) -> [MinTemp_Out]
  PCANB(BMS、DRIVE_MOTOR)/1(heatingctl) -> [HeatingCtl_Out]
  PCANB(BMS、DRIVE_MOTOR)/6(maxtemp) -> [MaxTemp_Out]
  PCANB(BMS、DRIVE_MOTOR)/7(maxcellvoltno) -> [MaxCellVoltNo_Out]
  PCANB(BMS、DRIVE_MOTOR)/8(mincellvoltno) -> [MinCellVoltNo_Out]
  PCANB(BMS、DRIVE_MOTOR)/9(mincellvolt) -> [MinCellVolt_Out]
  PCANB(BMS、DRIVE_MOTOR)/10(maxcellvolt) -> [MaxCellVolt_Out]
  [FunCall_50ms_Duty8] -> PCANB(BMS、DRIVE_MOTOR)/Trigger
  PCANB(BMS、DRIVE_MOTOR)/11(offChrRlyStr_Out) -> [offChrRlyStr_Out]
  PCANB(BMS、DRIVE_MOTOR)/18(OnChrRlyStr_Out) -> [OnChrRlyStr_Out]
  PCANB(BMS、DRIVE_MOTOR)/14(chrONCC_Out) -> [chrONCC_Out]
  PCANB(BMS、DRIVE_MOTOR)/15(chrOFFCC2_Out) -> [chrOFFCC2_Out]
  PCANB(BMS、DRIVE_MOTOR)/16(ChrCommunication_Out) -> [ChrCommunication_Out]
  PCANB(BMS、DRIVE_MOTOR)/19(PreRlyStr_Out) -> [PreRlyStr_Out]
  PCANB(BMS、DRIVE_MOTOR)/13(ChrReqVolt_Out) -> [ChrReqVolt_Out]
  PCANB(BMS、DRIVE_MOTOR)/21(PosRlyStr_Out) -> [PosRlyStr_Out]
  PCANB(BMS、DRIVE_MOTOR)/20(NegRlyStr_Out) -> [NegRlyStr_Out]
  PCANB(BMS、DRIVE_MOTOR)/17(ChrState_Out) -> [ChrState_Out]
  PCANB(BMS、DRIVE_MOTOR)/12(ChrReqCurr_Out) -> [ChrReqCurr_Out]
  PCANB(BMS、DRIVE_MOTOR)/24(MaxDisCurtLimit_Out) -> [MaxDisCurtLimit_Out]
  PCANB(BMS、DRIVE_MOTOR)/23(MaxChrPowerLimit_Out) -> [MaxChrPowerLimit_Out]
  PCANB(BMS、DRIVE_MOTOR)/25(MaxChrCurtLimit_Out) -> [MaxChrCurtLimit_Out]
  PCANB(BMS、DRIVE_MOTOR)/22(MaxDisPowerLimit_Out) -> [MaxDisPowerLimit_Out]
  PCANB(BMS、DRIVE_MOTOR)/26(Motor_Node) -> [Motor_Node]
  PCANB(BMS、DRIVE_MOTOR)/27(Motor_Current_Speed) -> [Motor_Current_Speed]
  PCANB(BMS、DRIVE_MOTOR)/38(ALM_BSU_FAULT_Out) -> [ALM_BSU_FAULT_Out]
  PCANB(BMS、DRIVE_MOTOR)/37(ALM_BSU_OFFLINE_Out) -> [ALM_BSU_OFFLINE_Out]
  PCANB(BMS、DRIVE_MOTOR)/39(ALM_BMU_FAIL_Out) -> [ALM_BMU_FAIL_Out]
  PCANB(BMS、DRIVE_MOTOR)/40(ALM_BATT_UC_Out) -> [ALM_BATT_UC_Out]
  PCANB(BMS、DRIVE_MOTOR)/36(ALM_CHRG_OCS_Out) -> [ALM_CHRG_OCS_Out]
  PCANB(BMS、DRIVE_MOTOR)/35(ALM_CHRG_OCT_Out) -> [ALM_CHRG_OCT_Out]
  PCANB(BMS、DRIVE_MOTOR)/41(ALM_BATT_OC_Out) -> [ALM_BATT_OC_Out]
  PCANB(BMS、DRIVE_MOTOR)/34(ALM_DSCH_OCS_Out) -> [ALM_DSCH_OCS_Out]
  PCANB(BMS、DRIVE_MOTOR)/42(ALM_AUX_FAIL_Out) -> [ALM_AUX_FAIL_Out]
  PCANB(BMS、DRIVE_MOTOR)/43(ALM_BATT_UV_Out) -> [ALM_BATT_UV_Out]
  PCANB(BMS、DRIVE_MOTOR)/33(ALM_DSCH_OCT_Out) -> [ALM_DSCH_OCT_Out]
  PCANB(BMS、DRIVE_MOTOR)/32(ALM_HALL_BREAK_Out) -> [ALM_HALL_BREAK_Out]
  PCANB(BMS、DRIVE_MOTOR)/44(ALM_BATT_OV_Out) -> [ALM_BATT_OV_Out]
  PCANB(BMS、DRIVE_MOTOR)/31(ALM_HVREL_FAIL_Out) -> [ALM_HVREL_FAIL_Out]
  PCANB(BMS、DRIVE_MOTOR)/45(ALM_BATT_DT_Out) -> [ALM_BATT_DT_Out]
  PCANB(BMS、DRIVE_MOTOR)/46(ALM_BATT_DV_Out) -> [ALM_BATT_DV_Out]
  PCANB(BMS、DRIVE_MOTOR)/30(ALM_LEAK_OC_Out) -> [ALM_LEAK_OC_Out]
  PCANB(BMS、DRIVE_MOTOR)/47(ALM_CELL_TBK_Out) -> [ALM_CELL_TBK_Out]
  PCANB(BMS、DRIVE_MOTOR)/29(ALM_PRECHRG_FAIL_Out) -> [ALM_PRECHRG_FAIL_Out]
  PCANB(BMS、DRIVE_MOTOR)/48(ALM_CELL_IBK_Out) -> [ALM_CELL_IBK_Out]
  PCANB(BMS、DRIVE_MOTOR)/28(ALM_VCU_OFFLINE_Out) -> [ALM_VCU_OFFLINE_Out]
  PCANB(BMS、DRIVE_MOTOR)/49(ALM_CELL_UT_Out) -> [ALM_CELL_UT_Out]
  PCANB(BMS、DRIVE_MOTOR)/50(ALM_CELL_OT_Out) -> [ALM_CELL_OT_Out]
  PCANB(BMS、DRIVE_MOTOR)/51(ALM_CELL_UV_Out) -> [ALM_CELL_UV_Out]
  PCANB(BMS、DRIVE_MOTOR)/52(ALM_CELL_OV_Out) -> [ALM_CELL_OV_Out]
  Subsystem1/1(Motec_Node) -> [Motec_Node]
  Function-Call Generator1/1 -> Subsystem1/Trigger
  Subsystem2/2(Fault) -> [Fault_Out]
  Subsystem2/3(operation_enable) -> [Operation_Enabled_Out]
  Subsystem2/4(quick_stop) -> [Quick_Stop_Out]
  Subsystem2/5(ready_switch_on) -> [Ready_Switch_On_Out]
  Subsystem2/6(switch_on_disable) -> [Switch_On_Disabled_Out]
  Subsystem2/7(switch_on) -> [Swtiched_On_Out]
  Subsystem2/8(target_reached) -> [Target_Reached_Out]
  Subsystem2/9(voltagle_enable) -> [Voltage_Enabled_Out]
  Subsystem2/10(warning_out) -> [Warning_Out]
  Subsystem2/1(Str_Status) -> [Str_Status]
  Function-Call Generator2/1 -> Subsystem2/Trigger
  PCANA(RES、AMI、MOTEC、BRAKE、STEER_SENSOR、IPC)/1(StrSr_Node) -> [StrSr_Node]
  PCANA(RES、AMI、MOTEC、BRAKE、STEER_SENSOR、IPC)/2(StrSr_Snr_Ang) -> [Str_Snr_Ang]
  PCANA(RES、AMI、MOTEC、BRAKE、STEER_SENSOR、IPC)/23(Brake_cmd_fault_flag_Out) -> [Brake_cmd_fault_flag_Out]
  PCANA(RES、AMI、MOTEC、BRAKE、STEER_SENSOR、IPC)/22(Brake_encoder_fault_sts_Out) -> [Brake_encoder_fault_sts_Out]
  PCANA(RES、AMI、MOTEC、BRAKE、STEER_SENSOR、IPC)/21(Brake_go_origin_over_flag_Out) -> [Brake_go_origin_over_flag_Out]
  PCANA(RES、AMI、MOTEC、BRAKE、STEER_SENSOR、IPC)/20(Brake_hd_fault_sts_Out) -> [Brake_hd_fault_sts_Out]
  PCANA(RES、AMI、MOTEC、BRAKE、STEER_SENSOR、IPC)/19(Brake_lowvolt_prtct_sts_Out) -> [Brake_lowvolt_prtct_sts_Out]
  PCANA(RES、AMI、MOTEC、BRAKE、STEER_SENSOR、IPC)/18(Brake_mtr_enable_flag_Out) -> Unit Delay1/1
  PCANA(RES、AMI、MOTEC、BRAKE、STEER_SENSOR、IPC)/17(Brake_mtr_origin_flag_Out) -> [Brake_mtr_origin_flag_Out]
  PCANA(RES、AMI、MOTEC、BRAKE、STEER_SENSOR、IPC)/16(Brake_mtr_stop_flag_Out) -> [Brake_mtr_stop_flag_Out]
  PCANA(RES、AMI、MOTEC、BRAKE、STEER_SENSOR、IPC)/15(Brake_offline_run_flag_O) -> [Brake_offline_run_flag_Out]
  PCANA(RES、AMI、MOTEC、BRAKE、STEER_SENSOR、IPC)/14(Brake_overcurrt_prtct_sts_Out) -> [Brake_overcurrt_prtct_sts_Out]
  PCANA(RES、AMI、MOTEC、BRAKE、STEER_SENSOR、IPC)/13(Brake_overheat_prtct_sts_Out) -> [Brake_overheat_prtct_sts_Out]
  PCANA(RES、AMI、MOTEC、BRAKE、STEER_SENSOR、IPC)/12(Brake_reg_rw_fault_flag_Out) -> [Brake_reg_rw_fault_flag_Out]
  PCANA(RES、AMI、MOTEC、BRAKE、STEER_SENSOR、IPC)/11(Brake_sensor1_sts_Out) -> [Brake_sensor1_sts_Out]
  PCANA(RES、AMI、MOTEC、BRAKE、STEER_SENSOR、IPC)/10(Brake_sensor2_sts_Out) -> [Brake_sensor2_sts_Out]
  PCANA(RES、AMI、MOTEC、BRAKE、STEER_SENSOR、IPC)/9(Brake_sensor3_sts_Out) -> [Brake_sensor3_sts_Out]
  PCANA(RES、AMI、MOTEC、BRAKE、STEER_SENSOR、IPC)/8(Brake_sensor4_sts_Out) -> [Brake_sensor4_sts_Out]
  PCANA(RES、AMI、MOTEC、BRAKE、STEER_SENSOR、IPC)/7(Brake_sensor5_sts_Out) -> [Brake_sensor5_sts_Out]
  PCANA(RES、AMI、MOTEC、BRAKE、STEER_SENSOR、IPC)/6(Brake_sensor6_sts_Out) -> [Brake_sensor6_sts_Out]
  PCANA(RES、AMI、MOTEC、BRAKE、STEER_SENSOR、IPC)/5(Brake_pos_enqual_Out) -> [Brake_pos_enqual_Out]
  PCANA(RES、AMI、MOTEC、BRAKE、STEER_SENSOR、IPC)/4(Brake_speed_enqual_Out) -> [Brake_speed_enqual_Out]
  PCANA(RES、AMI、MOTEC、BRAKE、STEER_SENSOR、IPC)/3(Brake_mtr_goalpos_Out) -> [Brake_mtr_goalpos_Out]
  PCANA(RES、AMI、MOTEC、BRAKE、STEER_SENSOR、IPC)/24(Brk_Node) -> [Brake_Node]
  Unit Delay1/1 -> [Brake_mtr_enable_flag_Out]
  PCANA(RES、AMI、MOTEC、BRAKE、STEER_SENSOR、IPC)/27(IPC_Acc) -> [IPC_Acc]
  PCANA(RES、AMI、MOTEC、BRAKE、STEER_SENSOR、IPC)/25(IPC_Steer) -> [IPC_Steer]
  PCANA(RES、AMI、MOTEC、BRAKE、STEER_SENSOR、IPC)/26(IPC_Brk) -> [IPC_Brk]
  PCANA(RES、AMI、MOTEC、BRAKE、STEER_SENSOR、IPC)/28(RES_Signal) -> [RES_SINGNAL]
  PCANB(BMS、DRIVE_MOTOR)/53(Str_UnderVolt_Warning_Out) -> [Str_UnderVolt_Warning_Out]
  PCANB(BMS、DRIVE_MOTOR)/54(Str_System_Error_Out) -> [Str_System_Error_Out]
  PCANB(BMS、DRIVE_MOTOR)/55(Str_Spd_Over_Alam_Out) -> [Str_Spd_Over_Alam_Out]
  PCANB(BMS、DRIVE_MOTOR)/56(Str_PwrMod_TempHigh_Warning_Out) -> [Str_PwrMod_TempHigh_Warning_Out]
  PCANB(BMS、DRIVE_MOTOR)/57(Str_PwrMod_TempHigh_Alarm_Out) -> [Str_PwrMod_TempHigh_Alarm_Out]
  PCANB(BMS、DRIVE_MOTOR)/58(Str_Para_Error_Out) -> [Str_Para_Error_Out]
  PCANB(BMS、DRIVE_MOTOR)/59(Str_Overvolt_Warning_Out) -> [Str_Overvolt_Warning_Out]
  PCANB(BMS、DRIVE_MOTOR)/62(Str_Over_PosError_Out) -> [Str_Over_PosError_Out]
  PCANB(BMS、DRIVE_MOTOR)/60(Str_Over_TopCurr_Out) -> [Str_Over_TopCurr_Out]
  PCANB(BMS、DRIVE_MOTOR)/63(Str_Limit_Pos_Alarm_Out) -> [Str_Limit_Pos_Alarm_Out]
  PCANB(BMS、DRIVE_MOTOR)/61(Str_Over_SpdError_Out) -> [Str_Over_SpdError_Out]
  PCANB(BMS、DRIVE_MOTOR)/67(Str_Encoder_Error_Out) -> [Str_Encoder_Error_Out]
  PCANB(BMS、DRIVE_MOTOR)/68(Str_Curr_Error_Fault_Out) -> [Str_Curr_Error_Fault_Out]
  PCANB(BMS、DRIVE_MOTOR)/64(Str_I2t_Warning_Out) -> [Str_I2t_Warning_Out]
  PCANB(BMS、DRIVE_MOTOR)/66(Str_Flash_Error_Out) -> [Str_Flash_Error_Out]
  PCANB(BMS、DRIVE_MOTOR)/65(Str_I2t_Alarm_Out) -> [Str_I2t_Alarm_Out]
  Unit Delay5/1 -> [AMI_State]
  PCANB(BMS、DRIVE_MOTOR)/69(AMI_State) -> Unit Delay5/1
  PCANB(BMS、DRIVE_MOTOR)/70(AMI_Node) -> [AMI_Node]
  [FunCall_10ms_Duty] -> PCANA(RES、AMI、MOTEC、BRAKE、STEER_SENSOR、IPC)/Trigger

== system FSAC2021_V1/VCU_KL_Read ==
  Read_VCU_AnaInput : Subsystem
  Read_VCU_DigInput : Subsystem
  Read_VCU_Freq(WheelSpeed) : Subsystem
  tag scope: ASMS=global, Acc_Lft_Disp_mv=global, Acc_Right_Disp_mv=global, Brake_Trigger=global, Compare_Volt_mv=global, EBS_GAS_Prs_1_mv=global, EBS_GAS_Prs_2_mv=global, EBS_Rel_Switch=global, FL_WhlSpd_Hz=global, FR_WhlSpd_Hz=global, HVMS=global, HV_LIGHT=global, LVMS=global, On_In_Switch=global, On_Out_Switch=global, RL_WhlSpd_Hz=global, RR_WhlSpd_Hz=global, START=global, liquid_Pressuress=global
  wires:
  [FunCall_50ms_Duty2] -> Read_VCU_Freq(WheelSpeed)/Trigger
  [FunCall_50ms_Duty6] -> Read_VCU_DigInput/Trigger
  [FunCall_50ms_Duty7] -> Read_VCU_AnaInput/Trigger
  Read_VCU_Freq(WheelSpeed)/1(RL_WhlSpd_Hz) -> [FL_WhlSpd_Hz], [RL_WhlSpd_Hz]
  Read_VCU_Freq(WheelSpeed)/2(RR_WhlSpd_Hz) -> [RR_WhlSpd_Hz], [FR_WhlSpd_Hz]
  Read_VCU_DigInput/1(LVMS) -> [LVMS]
  Read_VCU_DigInput/2(HVMS) -> [HVMS]
  Read_VCU_DigInput/3(ASMS) -> [ASMS]
  Read_VCU_DigInput/4(On_out_switch) -> [On_Out_Switch]
  Read_VCU_DigInput/5(Start) -> [START]
  Read_VCU_DigInput/6(On_in_switch) -> [On_In_Switch]
  Read_VCU_DigInput/7(HV_light) -> [HV_LIGHT]
  Read_VCU_DigInput/8(EBS_Rel) -> [EBS_Rel_Switch]
  Read_VCU_AnaInput/5(EBS_GAS2) -> [EBS_GAS_Prs_2_mv]
  Read_VCU_AnaInput/4(EBS_GAS1) -> [EBS_GAS_Prs_1_mv]
  Read_VCU_AnaInput/3(COMPARE_VOLTAGLE) -> [Compare_Volt_mv]
  Read_VCU_AnaInput/2(ACC_RIGHT) -> [Acc_Right_Disp_mv]
  Read_VCU_AnaInput/1(ACC_LEFT) -> [Acc_Lft_Disp_mv]
  Read_VCU_AnaInput/6(Brake_trigger) -> [Brake_Trigger]
  Read_VCU_AnaInput/7(liquid_presuress) -> [liquid_Pressuress]

== system FSAC2021_V1/CAN_SEND/(BRK、STR、DRIVER) ==
  BatVoltage_Out : Inport
  Motor_Current_Speed : Inport  Port=2
  ASSI_State : Inport  Port=3
  vspd : Inport  Port=4
  function : TriggerPort  TriggerType=function-call
  CANTransmit7 : ec55xxlib/RapidECU_U2/07CANCommucation/CANTransmit  canmodule=A  canbuffer=60  canmessageid=1161  canmessagetype=Standard(11-bit ID)  datalength=8  sampletime=-1
  MeaModule3 : ec55xxlib/RapidECU_U2/11Calibration/MeaModule  signal=To_AMI_OK
  MeaModule4 : ec55xxlib/RapidECU_U2/11Calibration/MeaModule  signal=Vspd
  MeaModule5 : ec55xxlib/RapidECU_U2/11Calibration/MeaModule  signal=Motor_Spd
  MeaModule6 : ec55xxlib/RapidECU_U2/11Calibration/MeaModule  signal=Voltage
  MeaModule7 : ec55xxlib/RapidECU_U2/11Calibration/MeaModule  signal=ASSI_state
  Terminator7 : Terminator
  To_AMI : Subsystem
  wires:
  To_AMI/1(output) -> CANTransmit7/1
  CANTransmit7/1 -> MeaModule3/1
  BatVoltage_Out/1 -> MeaModule6/1
  Motor_Current_Speed/1 -> MeaModule5/1
  ASSI_State/1 -> MeaModule7/1
  vspd/1 -> MeaModule4/1
  MeaModule3/1 -> Terminator7/1
  MeaModule4/1 -> To_AMI/1(vspd_in)
  MeaModule5/1 -> To_AMI/2(mtr_rpm_in)
  MeaModule6/1 -> To_AMI/3(Battery_Volt_in)
  MeaModule7/1 -> To_AMI/4(assi_status_in)

== system FSAC2021_V1/CAN_SEND/Subsystem1 ==
  Tmt_RPD01_CAN_FunCall : Inport
  Switch_On_Ctrl : Inport  Port=2
  Enable_Voltage_Ctrl : Inport  Port=3
  Quick_Stop_Ctrl : Inport  Port=4
  Enable_Operation_Ctrl : Inport  Port=5
  New_Set_Point_Ctrl : Inport  Port=6
  Abs_or_Rel_Ctrl : Inport  Port=7
  Halt_Ctrl : Inport  Port=8
  Position_set : Inport  Port=9
  Tmt_NMT_CAN_FunCall : Inport  Port=10
  NMT_nodeorder : Inport  Port=11
  NMT_nodectrl : Inport  Port=12
  Tmt_SDO_CAN_FunCall : Inport  Port=13
  Encoder_Msg_Data : Inport  Port=14
  Fault_Reset : Inport  Port=15
  ASSI_STATE : Inport  Port=16
  Brk_Mtr_Enbale : Subsystem  TreatAsAtomicUnit=on
  CANTransmit : ec55xxlib/RapidECU_U2/07CANCommucation/CANTransmit  canmodule=A  canbuffer=63  canmessageid=513  canmessagetype=Standard(11-bit ID)  datalength=6  sampletime=-1
  CANTransmit1 : ec55xxlib/RapidECU_U2/07CANCommucation/CANTransmit  canmodule=A  canbuffer=62  canmessageid=0  canmessagetype=Standard(11-bit ID)  datalength=2  sampletime=-1
  CANTransmit2 : ec55xxlib/RapidECU_U2/07CANCommucation/CANTransmit  canmodule=A  canbuffer=61  canmessageid=1537  canmessagetype=Standard(11-bit ID)  datalength=6  sampletime=-1
  Compare To Constant : simulink/Logic and Bit Operations/Compare To Constant  relop=>=  const=3  OutDataTypeStr=boolean
  Constant : Constant  Value=0  OutDataTypeStr=uint8
  Data Type Conversion{,1..16} (17 alike) : DataTypeConversion
  Demux : Demux  Outputs=6
  MOTEC_CONTROL : Subsystem
  MOTEC_ENCODER1 : Subsystem
  MOTEC_NMT : Subsystem
  MeaModule10 : ec55xxlib/RapidECU_U2/11Calibration/MeaModule  signal=ENCODER_SEND
  MeaModule8 : ec55xxlib/RapidECU_U2/11Calibration/MeaModule  signal=Metoc_Move
  MeaModule9 : ec55xxlib/RapidECU_U2/11Calibration/MeaModule  signal=MNT_SEND
  Switch : Switch  Criteria=u2 > Threshold
  Terminator : Terminator
  Terminator1 : Terminator
  Terminator2 : Terminator
  Unit Delay{,1..17} (18 alike) : UnitDelay  SampleTime=-1
  wires:
  CANTransmit/1 -> MeaModule8/1
  Halt_Ctrl/1 -> Unit Delay7/1
  Unit Delay3/1 -> Data Type Conversion5/1
  Unit Delay4/1 -> Data Type Conversion6/1
  Unit Delay5/1 -> Data Type Conversion7/1
  Unit Delay2/1 -> Data Type Conversion4/1
  Quick_Stop_Ctrl/1 -> Unit Delay2/1
  Abs_or_Rel_Ctrl/1 -> Unit Delay5/1
  New_Set_Point_Ctrl/1 -> Unit Delay4/1
  Enable_Voltage_Ctrl/1 -> Unit Delay1/1
  Enable_Operation_Ctrl/1 -> Unit Delay3/1
  Unit Delay1/1 -> Data Type Conversion3/1
  Unit Delay8/1 -> Data Type Conversion10/1
  Unit Delay7/1 -> Data Type Conversion9/1
  Switch_On_Ctrl/1 -> Unit Delay/1
  Unit Delay/1 -> Data Type Conversion2/1
  Data Type Conversion13/1 -> Unit Delay13/1
  Data Type Conversion12/1 -> Unit Delay12/1
  NMT_nodectrl/1 -> Unit Delay9/1
  Data Type Conversion/1 -> MOTEC_NMT/1(NMT_nodeorder_in)
  NMT_nodeorder/1 -> Unit Delay10/1
  Tmt_NMT_CAN_FunCall/1 -> MOTEC_NMT/Trigger
  Data Type Conversion1/1 -> MOTEC_NMT/2(NMT_nodectrl_in)
  CANTransmit1/1 -> MeaModule9/1
  Tmt_SDO_CAN_FunCall/1 -> MOTEC_ENCODER1/Trigger
  Encoder_Msg_Data/1 -> Demux/1
  Data Type Conversion16/1 -> Unit Delay16/1
  Unit Delay9/1 -> Data Type Conversion1/1
  Unit Delay10/1 -> Data Type Conversion/1
  Data Type Conversion14/1 -> Unit Delay14/1
  Demux/5 -> Data Type Conversion15/1
  CANTransmit2/1 -> MeaModule10/1
  Unit Delay6/1 -> Data Type Conversion8/1
  Data Type Conversion8/1 -> MOTEC_CONTROL/1(Fault_Reset_in)
  Data Type Conversion10/1 -> MOTEC_CONTROL/2(Position_set_in)
  Data Type Conversion3/1 -> MOTEC_CONTROL/8(Enable_Voltage_Ctrl_in)
  Data Type Conversion4/1 -> MOTEC_CONTROL/7(Quick_Stop_Ctrl_in)
  Data Type Conversion5/1 -> MOTEC_CONTROL/9(Enable_Operation_Ctrl_in)
  Position_set/1 -> Unit Delay8/1
  Data Type Conversion7/1 -> MOTEC_CONTROL/5(Abs_or_Rel_Ctrl_in)
  Data Type Conversion6/1 -> MOTEC_CONTROL/3(New_Pos_Set_in)
  Data Type Conversion2/1 -> MOTEC_CONTROL/6(Switch_On_Ctrl_in)
  Data Type Conversion9/1 -> MOTEC_CONTROL/4(Halt_Ctrl_in)
  Tmt_RPD01_CAN_FunCall/1 -> MOTEC_CONTROL/Trigger
  Demux/4 -> Data Type Conversion14/1
  MeaModule8/1 -> Terminator/1
  Data Type Conversion15/1 -> Unit Delay15/1
  Demux/6 -> Data Type Conversion16/1
  Demux/2 -> Data Type Conversion12/1
  MeaModule9/1 -> Terminator1/1
  Fault_Reset/1 -> Unit Delay6/1
  Data Type Conversion11/1 -> Unit Delay11/1
  Demux/1 -> Data Type Conversion11/1
  Demux/3 -> Data Type Conversion13/1
  MeaModule10/1 -> Terminator2/1
  MOTEC_CONTROL/1(output) -> CANTransmit/1
  MOTEC_NMT/1(output) -> CANTransmit1/1
  MOTEC_ENCODER1/1(output) -> CANTransmit2/1
  Unit Delay11/1 -> MOTEC_ENCODER1/1(Str_Encoder1_in)
  Unit Delay12/1 -> MOTEC_ENCODER1/2(Str_Encoder2_in)
  Unit Delay14/1 -> MOTEC_ENCODER1/4(Str_Encoder4_in)
  Unit Delay13/1 -> MOTEC_ENCODER1/3(Str_Encoder3_in)
  Unit Delay16/1 -> MOTEC_ENCODER1/6(Str_Encoder6_in)
  ASSI_STATE/1 -> Compare To Constant/1
  Compare To Constant/1 -> Switch/2
  Unit Delay15/1 -> Switch/3
  Switch/1 -> MOTEC_ENCODER1/5(Str_Encoder5_in)
  Constant/1 -> Unit Delay17/1
  Unit Delay17/1 -> Switch/1
